simulink model "Demo_MPC_Laguerre"  (R2020a)
settings: Solver=VariableStepAuto  StartTime=0.0  StopTime=10.0  FixedStep=0.01  RelTol=1e-3
settings Model: Creator=86150  LastModifiedBy=86150

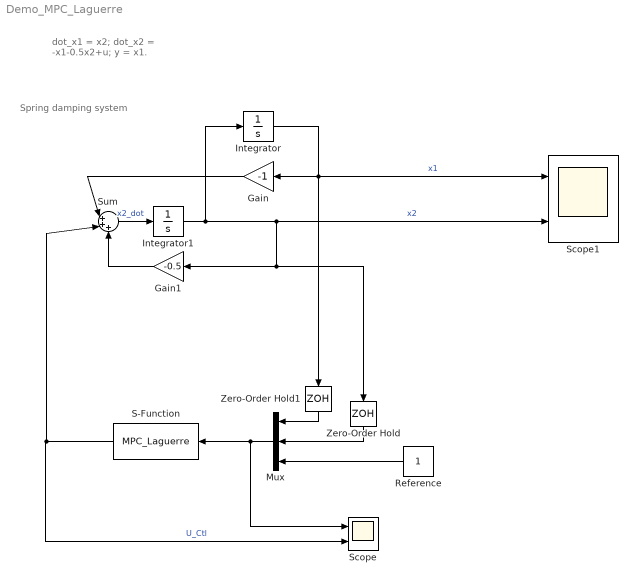
== system Demo_MPC_Laguerre ==
  note: dot_x1 = x2;
      | dot_x2 = -x1-0.5x2+u;
      | y = x1.
  note: Spring damping system
  Gain : Gain  Gain=-1
  Gain1 : Gain  Gain=-0.5
  Integrator : Integrator
  Integrator1 : Integrator
  Mux : Mux  Inputs=3
  Reference : Constant
  S-Function : S-Function  FunctionName=MPC_Laguerre  SFunctionDeploymentMode=off  EnableBusSupport=off
  Scope : Scope  NumInputPorts=2
  Scope1 : Scope  NumInputPorts=2
  Sum : Sum  Inputs=|+++
  Zero-Order Hold : ZeroOrderHold  SampleTime=0.001
  Zero-Order Hold1 : ZeroOrderHold  SampleTime=0.001
  wires:
  Mux/1 -> Scope/1, S-Function/1
  Reference/1 -> Mux/3
  S-Function/1 -> Sum/2, Scope/2  "U_Ctl"
  Zero-Order Hold/1 -> Mux/2
  Zero-Order Hold1/1 -> Mux/1
  Integrator/1 -> Zero-Order Hold1/1, Gain/1, Scope1/1  "x1"
  Sum/1 -> Integrator1/1  "x2_dot"
  Gain/1 -> Sum/1
  Gain1/1 -> Sum/3
  Integrator1/1 -> Integrator/1, Zero-Order Hold/1, Gain1/1, Scope1/2  "x2"
